simulink model "lab9"  (R2023b)
settings: Solver=ode45  StartTime=0.0  StopTime=150.0  MaxStep=0.05  RelTol=1e-3
libraries: simulink x1
settings Model: Creator=insomnia  LastModifiedBy=insomnia

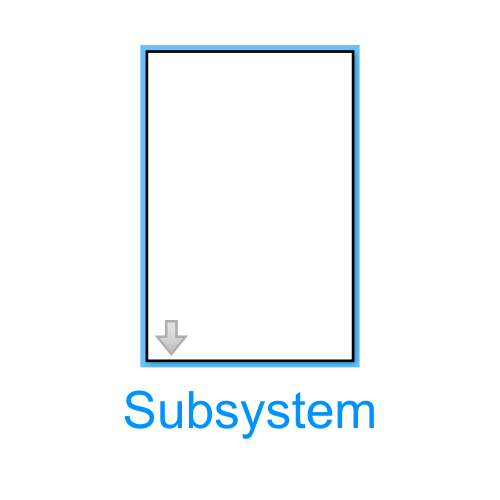
[thumbnail: Simulink's stored preview of the top-level diagram]
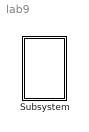
== system lab9 ==
  Subsystem : Subsystem  mask{h1=4, h2=2, S1=1, S2=2, Swy1=0.2, Swy2=0.2, fi1=1, fi2=1, g=9.81, Qwe=2}

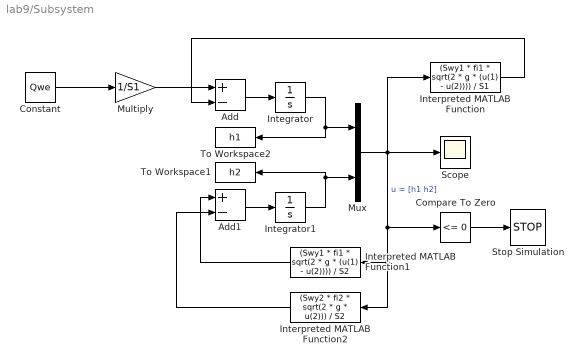
== system lab9/Subsystem ==
  Add : Sum  Inputs=+-
  Add1 : Sum  Inputs=+-
  Compare To Zero : simulink/Logic and Bit Operations/Compare To Zero  relop=<=  OutDataTypeStr=boolean
  Constant : Constant  Value=Qwe
  Integrator : Integrator  InitialCondition=h1
  Integrator1 : Integrator  InitialCondition=h2
  Interpreted MATLAB Function : MATLABFcn  MATLABFcn=(Swy1 * fi1 * sqrt(2 * g * (u(1) - u(2)))) / S1
  Interpreted MATLAB Function1 : MATLABFcn  MATLABFcn=(Swy1 * fi1 * sqrt(2 * g * (u(1) - u(2)))) / S2
  Interpreted MATLAB Function2 : MATLABFcn  MATLABFcn=(Swy2 * fi2 * sqrt(2 * g * u(2))) / S2
  Multiply : Gain  Gain=1/S1
  Mux : Mux  Inputs=2
  Scope : Scope
  Stop Simulation : Stop
  To Workspace1 : ToWorkspace  VariableName=h2  SampleTime=-1
  To Workspace2 : ToWorkspace  VariableName=h1  SampleTime=-1
  wires:
  Multiply/1 -> Add/1
  Constant/1 -> Multiply/1
  Add/1 -> Integrator/1
  Integrator/1 -> To Workspace2/1, Mux/1
  Integrator1/1 -> To Workspace1/1, Mux/2
  Add1/1 -> Integrator1/1
  Mux/1 -> Compare To Zero/1, Interpreted MATLAB Function2/1, Interpreted MATLAB Function1/1, Interpreted MATLAB Function/1, Scope/1  "u = [h1 h2]"
  Interpreted MATLAB Function/1 -> Add/2
  Interpreted MATLAB Function1/1 -> Add1/1
  Interpreted MATLAB Function2/1 -> Add1/2
  Compare To Zero/1 -> Stop Simulation/1
